simulink model "DCmotor"  (R2020a)
settings: Solver=VariableStepAuto  StartTime=0.0  StopTime=10  RelTol=1e-3
values from neighbouring files (symbols this model uses):
  B = 0.010    (= 0.01)    [DCmotor_parameters.m]
  Bl = 0.02    [DCmotor_parameters.m]
  J = 0.010    (= 0.01)    [DCmotor_parameters.m]
  Jl = 0.03    [DCmotor_parameters.m]
  Ke = 2    [DCmotor_parameters.m]
  Km = 2    [DCmotor_parameters.m]
  L = 0.0025    [DCmotor_parameters.m]
  N = 1    [DCmotor_parameters.m]
  R = 0.434    [DCmotor_parameters.m]
settings Model: Creator=riccardo  LastModifiedBy=giovanni

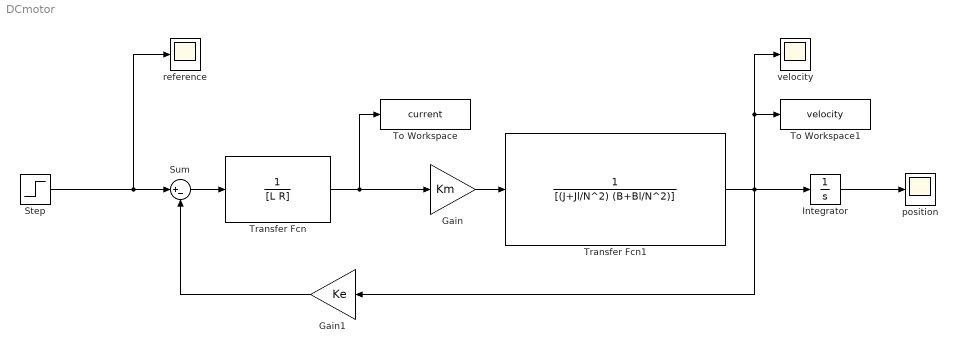
== system DCmotor ==
  Gain : Gain  Gain=Km
  Gain1 : Gain  Gain=Ke
  Integrator : Integrator
  Step : Step  After=10  SampleTime=0
  Sum : Sum  Inputs=|+-
  To Workspace : ToWorkspace  VariableName=current  SaveFormat=Timeseries  SampleTime=-1
  To Workspace1 : ToWorkspace  VariableName=velocity  SaveFormat=Timeseries  SampleTime=-1
  Transfer Fcn : TransferFcn  Denominator=[L R]
  Transfer Fcn1 : TransferFcn  Denominator=[(J+Jl/N^2) (B+Bl/N^2)]
  position : Scope
  reference : Scope
  velocity : Scope
  wires:
  Sum/1 -> Transfer Fcn/1
  Transfer Fcn/1 -> Gain/1, To Workspace/1
  Transfer Fcn1/1 -> Gain1/1, velocity/1, To Workspace1/1, Integrator/1
  Gain1/1 -> Sum/2
  Integrator/1 -> position/1
  Gain/1 -> Transfer Fcn1/1
  Step/1 -> reference/1, Sum/1
